simulink model "subsys"  (Simulink 7.9)
settings: Solver=ode45  StartTime=0.0  StopTime=10.0  RelTol=1e-3
settings Model: Creator=Nice  LastModifiedBy=Nice

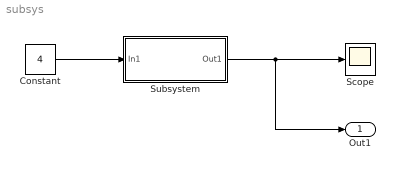
== system subsys ==
  Constant : Constant  Value=4
  Scope : Scope
  Subsystem : Subsystem
  Out1 : Outport
  wires:
  Constant/1 -> Subsystem/1(In1)
  Subsystem/1(Out1) -> Scope/1, Out1/1

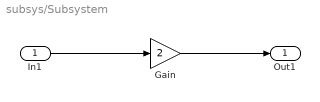
== system subsys/Subsystem ==
  In1 : Inport
  Gain : Gain  Gain=2
  Out1 : Outport
  wires:
  In1/1 -> Gain/1
  Gain/1 -> Out1/1
